simulink model "Motor_Control"  (R2020b)
settings: Solver=VariableStepAuto  StartTime=0.0  StopTime=12  RelTol=1e-3
model workspace (MAT data in the model file):
  value = 1
settings Model: Creator=lenovo  LastModifiedBy=lenovo

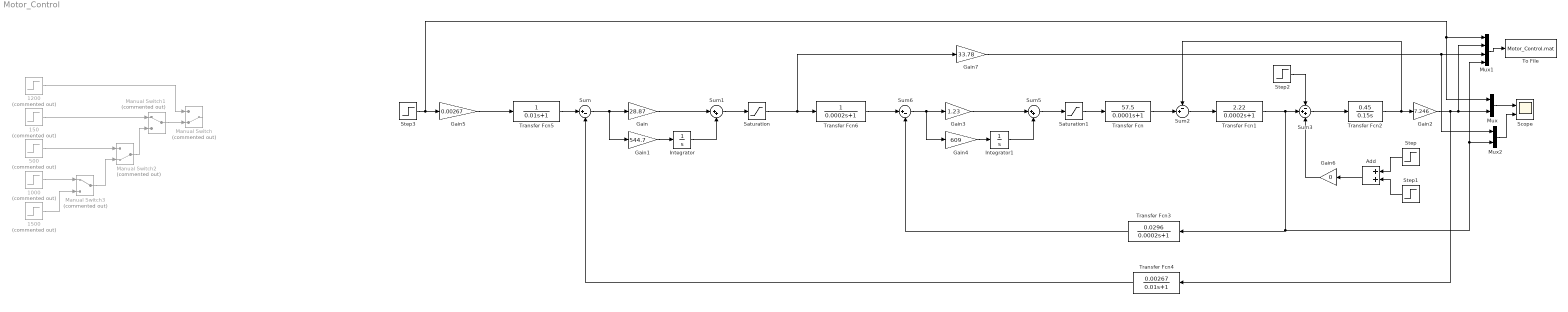
== system Motor_Control ==
  1000 : Step  Commented=on  After=1000  SampleTime=0
  1200 : Step  Commented=on  After=1200  SampleTime=0
  150 : Step  Commented=on  After=150  SampleTime=0
  1500 : Step  Commented=on  After=1500  SampleTime=0
  500 : Step  Commented=on  After=500  SampleTime=0
  Add : Sum
  Gain : Gain  Gain=28.87
  Gain1 : Gain  Gain=544.7
  Gain2 : Gain  Gain=7.246
  Gain3 : Gain  Gain=1.23
  Gain4 : Gain  Gain=609
  Gain5 : Gain  Gain=0.00267
  Gain6 : Gain  Gain=0
  Gain7 : Gain  Gain=33.78
  Integrator : Integrator  LimitOutput=on  UpperSaturationLimit=4  LowerSaturationLimit=-4
  Integrator1 : Integrator  LimitOutput=on  UpperSaturationLimit=4  LowerSaturationLimit=-4
  Manual Switch : ManualSwitch  Commented=on  CurrentSetting=0
  Manual Switch1 : ManualSwitch  Commented=on
  Manual Switch2 : ManualSwitch  Commented=on  CurrentSetting=0
  Manual Switch3 : ManualSwitch  Commented=on
  Mux : Mux  Inputs=2
  Mux1 : Mux
  Mux2 : Mux  Inputs=2
  Saturation : Saturate  UpperLimit=4  LowerLimit=0
  Saturation1 : Saturate  UpperLimit=4  LowerLimit=0
  Scope : Scope  NumInputPorts=2
  Step : Step  Time=5  After=5  SampleTime=0
  Step1 : Step  Time=6  After=-5  SampleTime=0
  Step2 : Step  After=90  SampleTime=0
  Step3 : Step  After=1500  SampleTime=0
  Sum : Sum  Inputs=|+-
  Sum1 : Sum  Inputs=|++
  Sum2 : Sum  Inputs=-+|
  Sum3 : Sum  Inputs=-++
  Sum5 : Sum  Inputs=|++
  Sum6 : Sum  Inputs=|+-
  To File : ToFile  Filename=Motor_Control.mat  MatrixName=motor_response
  Transfer Fcn : TransferFcn  Numerator=[57.5]  Denominator=[0.0001 1]
  Transfer Fcn1 : TransferFcn  Numerator=[2.22]  Denominator=[0.0002 1]
  Transfer Fcn2 : TransferFcn  Numerator=[0.45]  Denominator=[0.15 0]
  Transfer Fcn3 : TransferFcn  Numerator=[0.0296]  Denominator=[0.0002 1]
  Transfer Fcn4 : TransferFcn  Numerator=[0.00267]  Denominator=[0.01 1]
  Transfer Fcn5 : TransferFcn  Denominator=[0.01 1]
  Transfer Fcn6 : TransferFcn  Denominator=[0.0002 1]
  wires:
  Sum/1 -> Gain1/1, Gain/1
  Gain1/1 -> Integrator/1
  Gain/1 -> Sum1/1
  Integrator/1 -> Sum1/2
  Sum1/1 -> Saturation/1
  Sum3/1 -> Transfer Fcn2/1
  Transfer Fcn2/1 -> Sum2/1, Gain2/1
  Gain2/1 -> Transfer Fcn4/1, Mux1/2, Mux/2
  Transfer Fcn/1 -> Sum2/2
  Sum2/1 -> Transfer Fcn1/1
  Gain4/1 -> Integrator1/1
  Saturation1/1 -> Transfer Fcn/1
  Integrator1/1 -> Sum5/2
  Sum5/1 -> Saturation1/1
  Sum6/1 -> Gain4/1, Gain3/1
  Gain3/1 -> Sum5/1
  Transfer Fcn3/1 -> Sum6/2
  Transfer Fcn4/1 -> Sum/2
  Transfer Fcn5/1 -> Sum/1
  Saturation/1 -> Gain7/1, Transfer Fcn6/1
  Transfer Fcn6/1 -> Sum6/1
  Step2/1 -> Sum3/1
  Gain5/1 -> Transfer Fcn5/1
  1200/1 -> Manual Switch/1
  Manual Switch1/1 -> Manual Switch/2
  150/1 -> Manual Switch1/1
  Manual Switch2/1 -> Manual Switch1/2
  500/1 -> Manual Switch2/1
  Manual Switch3/1 -> Manual Switch2/2
  1000/1 -> Manual Switch3/1
  1500/1 -> Manual Switch3/2
  Gain6/1 -> Sum3/3
  Add/1 -> Gain6/1
  Step/1 -> Add/1
  Step1/1 -> Add/2
  Transfer Fcn1/1 -> Mux2/2, Mux1/4, Transfer Fcn3/1, Sum3/2
  Mux/1 -> Scope/1
  Mux1/1 -> To File/1
  Step3/1 -> Mux/1, Mux1/1, Gain5/1
  Gain7/1 -> Mux2/1, Mux1/3
  Mux2/1 -> Scope/2
